simulink model "ComparativoModelodeControle"  (R2021a)
settings: Solver=VariableStepAuto  StartTime=0.0  StopTime=450  RelTol=1e-3
settings Model: Creator=Usuario  LastModifiedBy=Usuario

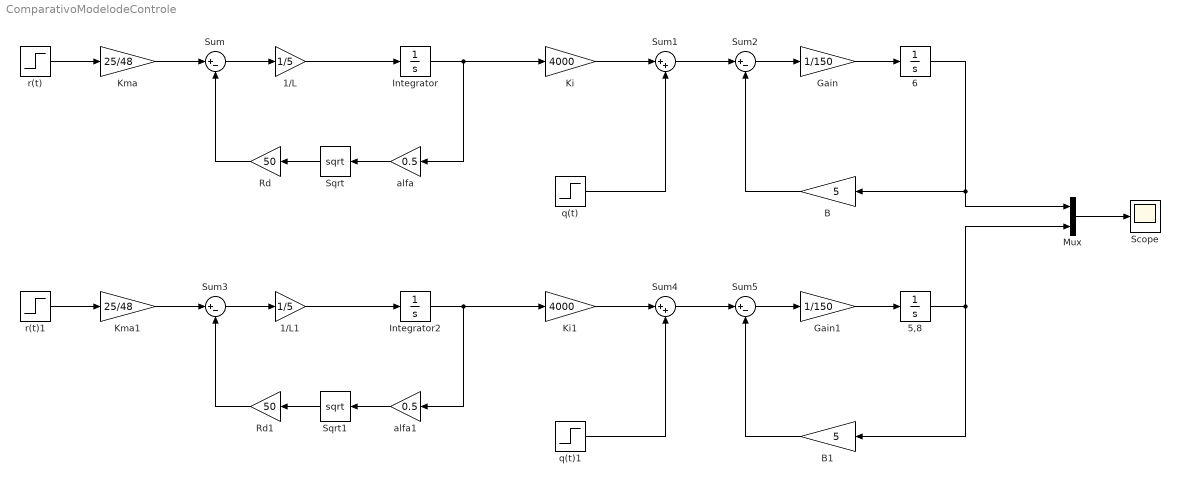
== system ComparativoModelodeControle ==
  1/L : Gain  Gain=1/5
  1/L1 : Gain  Gain=1/5
  5,8 : Integrator
  6 : Integrator
  B : Gain  Gain=5
  B1 : Gain  Gain=5
  Gain : Gain  Gain=1/150
  Gain1 : Gain  Gain=1/150
  Integrator : Integrator
  Integrator2 : Integrator
  Ki : Gain  Gain=4000
  Ki1 : Gain  Gain=4000
  Kma : Gain  Gain=25/48
  Kma1 : Gain  Gain=25/48
  Mux : Mux  Inputs=2
  Rd : Gain  Gain=50
  Rd1 : Gain  Gain=50
  Scope : Scope
  Sqrt : Sqrt  SaturateOnIntegerOverflow=on
  Sqrt1 : Sqrt  SaturateOnIntegerOverflow=on
  Sum{,2..3,5} (4 alike) : Sum  Inputs=|+-
  Sum1 : Sum  Inputs=|++
  Sum4 : Sum  Inputs=|++
  alfa : Gain  Gain=0.5
  alfa1 : Gain  Gain=0.5
  q(t) : Step  Time=0  After=0  SampleTime=0
  q(t)1 : Step  Time=0  After=0  SampleTime=0
  r(t) : Step  Time=200  Before=5.76  After=6  SampleTime=0
  r(t)1 : Step  Time=200  Before=5.76  After=5.8  SampleTime=0
  wires:
  Kma/1 -> Sum/1
  Sum/1 -> 1/L/1
  1/L/1 -> Integrator/1
  Rd/1 -> Sum/2
  Sqrt/1 -> Rd/1
  alfa/1 -> Sqrt/1
  Integrator/1 -> Ki/1, alfa/1
  Ki/1 -> Sum1/1
  q(t)/1 -> Sum1/2
  Sum1/1 -> Sum2/1
  Sum2/1 -> Gain/1
  Gain/1 -> 6/1
  B/1 -> Sum2/2
  6/1 -> Mux/1, B/1
  r(t)/1 -> Kma/1
  5,8/1 -> Mux/2, B1/1
  q(t)1/1 -> Sum4/2
  Gain1/1 -> 5,8/1
  B1/1 -> Sum5/2
  Ki1/1 -> Sum4/1
  Sum5/1 -> Gain1/1
  Sum4/1 -> Sum5/1
  alfa1/1 -> Sqrt1/1
  Integrator2/1 -> Ki1/1, alfa1/1
  Rd1/1 -> Sum3/2
  Sum3/1 -> 1/L1/1
  Kma1/1 -> Sum3/1
  r(t)1/1 -> Kma1/1
  1/L1/1 -> Integrator2/1
  Sqrt1/1 -> Rd1/1
  Mux/1 -> Scope/1
